simulink model "feedback"  (R2016a)
settings: Solver=FixedStepDiscrete  StartTime=0.0  StopTime=10.0  RelTol=1e-3
libraries: rvs x11
settings Model: Creator=Arthur  LastModifiedBy=arthur
settings DataIOCC: LimitDataPoints=on  SaveFormat=Array
settings DebuggingCC: SolverPrmCheckMsg=warning
settings HardwareCC: ProdBitPerPointer=32  ProdLargestAtomicFloat=None  ProdIntDivRoundTo=Undefined  ProdEndianess=Unspecified  ProdWordSize=32  ProdHWDeviceType=32-bit Generic
settings ModelReferenceCC: PropagateSignalLabelsOutOfModel=off
settings ConfigComp: CovModelRefEnable=Off  CovSFcnEnable=off

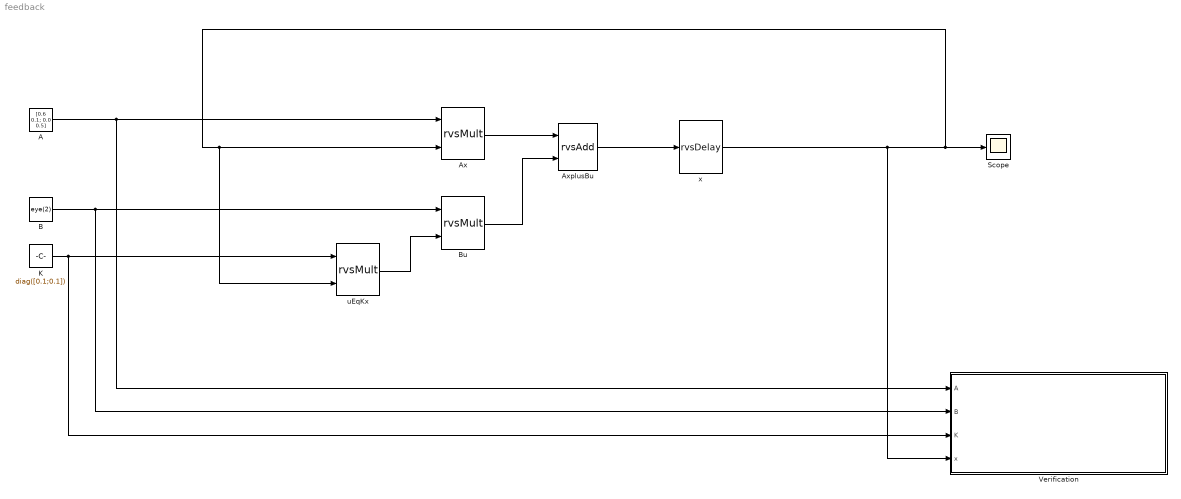
== system feedback ==
  A : Constant  Value=[0.6 0.1; 0.0 0.5]
  Ax : rvs/rvsMult
  AxplusBu : rvs/rvsAdd
  B : Constant  Value=eye(2)
  Bu : rvs/rvsMult
  K : Constant  Value=diag([0.1;0.1])
  Scope : Scope
  Verification : Subsystem
  uEqKx : rvs/rvsMult
  x : rvs/rvsDelay  xInit=[0.7;-0.5]
  wires:
  Ax/1 -> AxplusBu/1
  Bu/1 -> AxplusBu/2
  uEqKx/1 -> Bu/2
  AxplusBu/1 -> x/1
  A/1 -> Verification/1(A), Ax/1
  B/1 -> Verification/2(B), Bu/1
  x/1 -> Verification/4(x), Scope/1, uEqKx/2, Ax/2
  K/1 -> Verification/3(K), uEqKx/1

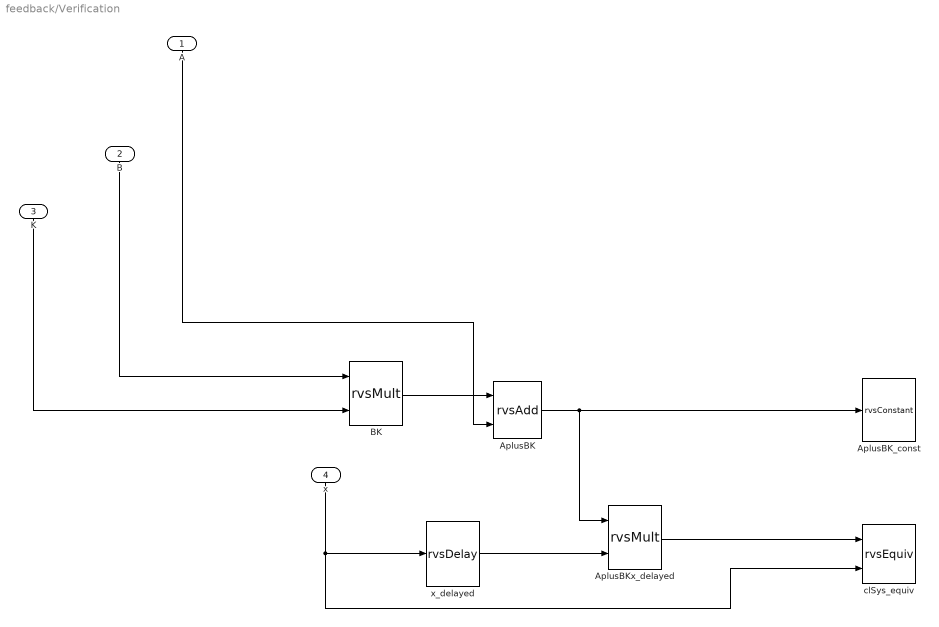
== system feedback/Verification ==
  A : Inport
  B : Inport  Port=2
  K : Inport  Port=3
  x : Inport  Port=4
  AplusBK : rvs/rvsAdd
  AplusBK_const : rvs/rvsConstant
  AplusBKx_delayed : rvs/rvsMult
  BK : rvs/rvsMult
  clSys_equiv : rvs/rvsEquiv  tol=1e-9  nIgnoreSteps=1
  x_delayed : rvs/rvsDelay  xInit=[0]
  wires:
  A/1 -> AplusBK/2
  B/1 -> BK/1
  K/1 -> BK/2
  BK/1 -> AplusBK/1
  AplusBK/1 -> AplusBKx_delayed/1, AplusBK_const/1
  x_delayed/1 -> AplusBKx_delayed/2
  AplusBKx_delayed/1 -> clSys_equiv/1
  x/1 -> clSys_equiv/2, x_delayed/1
